simulink model "Turbine_State_Machine_Testrig_org"  (Simulink 10.0)
settings: Solver=ode45  StartTime=0.0  StopTime=20  MaxStep=1e-4  RelTol=1e-3  EnableMultiTasking=on
undefined symbols (not defined in the file): sigbuilder_block
libraries: Turbine_State_Machine_Lib x1
Description:
  | Copyright 2009-2017 The MathWorks, Inc. MathWorks, Inc.
settings Model: Creator=smiller  LastModifiedBy=bhisma
settings DataIOCC: LimitDataPoints=on  SignalLoggingSaveFormat=ModelDataLogs
settings OptimizationCC: ExpressionDepthLimit=2147483647
settings DebuggingCC: FcnCallInpInsideContextMsg=warning  AllowSymbolicDim=off  StateNameClashWarn=warning
settings SFSimCC: SimParseCustomCode=off
settings GRTTargetCC: GeneratePreprocessorConditionals=Disable all
settings ConfigComp: CovExternalEMLEnable=off  CovSFcnEnable=off

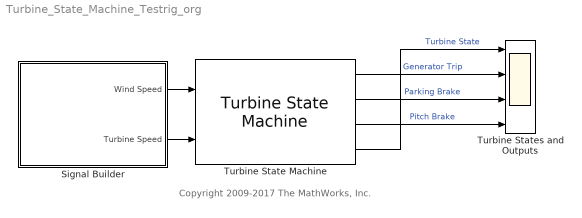
== system Turbine_State_Machine_Testrig_org ==
  note: Copyright 2009-2017 The MathWorks, Inc.
  Signal Builder : Subsystem  Tag=STV Subsys  LoadFcn=sigbuilder_block('load');  StartFcn=sigbuilder_block('start');  StopFcn=sigbuilder_block('stop');  ClipboardFcn=sigbuilder_block('clipboard');  mask(Sigbuilder block){tuvar=[0:10]}
      mask help: Sigbuilder GUI
      mask init:
      | if ~strcmp(get_param(bdroot(gcbh),'SimulationStatus'),'stopped') tuvar = sigbuilder_block('maskInit'); end
      settings: CopyFcn=sigbuilder_block('copy');  DeleteFcn=sigbuilder_block('delete');  ModelCloseFcn=sigbuilder_block('modelClose');  PreSaveFcn=sigbuilder_block('preSave');  PauseFcn=sigbuilder_block('pause')  ContinueFcn=sigbuilder_block('continue')  NameChangeFcn=sigbuilder_block('namechange');  OpenFcn=sigbuilder_block('open',[3 32.25 762 490.5 ]);  CloseFcn=sigbuilder_block('close');
      mask Display: plot(0, 0, 100, 100,[2, 2, 32, 32, 2], [68, 8, 8, 68, 68],[32, 2], [38, 38], [32, 19, 2],[53, 60, 44], [32, 17, 17, 2],[16, 16, 31, 31]);txt = getActiveGroup(gcbh);text(2, 100, txt,'verticalAlignment', 'top');
  Turbine State Machine : Turbine_State_Machine_Lib/Turbine State Machine
  Turbine States and Outputs : Scope  NumInputPorts=4
  wires:
  Turbine State Machine/4 -> Turbine States and Outputs/1  "Turbine State"
  Signal Builder/1(Wind Speed) -> Turbine State Machine/1
  Signal Builder/2(Turbine Speed) -> Turbine State Machine/2
  Turbine State Machine/1 -> Turbine States and Outputs/2  "Generator Trip"
  Turbine State Machine/2 -> Turbine States and Outputs/3  "Parking Brake"
  Turbine State Machine/3 -> Turbine States and Outputs/4  "Pitch Brake"

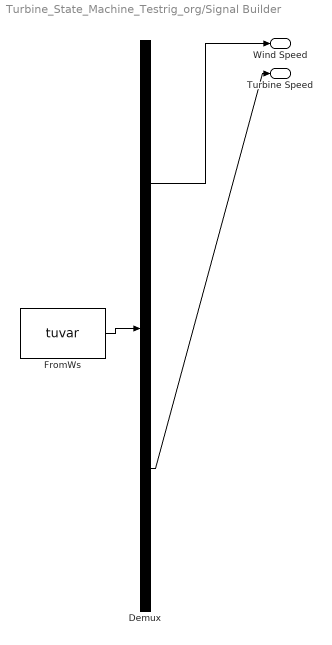
== system Turbine_State_Machine_Testrig_org/Signal Builder ==
  Demux : Demux  Tag=STV Demux  Outputs=2
  FromWs : FromWorkspace  Tag=STV FromWs  VariableName=tuvar  SampleTime=0  SigBuilderData=DataTag0  VnvData=DataTag1
      SigBuilderData=|
      | common.afterFinalStr = 'Extrapolate'
      | common.sampleTime = 0
      | dataSet(1).timeRange = [0 20]
      | dataSet(1).name = 'Simple Start and Stop'
      | dataSet(2).timeRange = [0 20]
      | dataSet(2).name = 'High Winds'
      | dataSet(3).timeRange = [0 20]
      | dataSet(3).name = 'Turbine Overspeed'
      | sbobj.Groups(1).Name = 'Simple Start and Stop'
      | sbobj.Groups(1).Signals(1).Name = 'Wind Speed'
      | sbobj.Groups(1).Signals(1).XData = [0 6 8.66 14 20]
      | sbobj.Groups(1).Signals(1).YData = [0 10 10 0 0]
      | sbobj.Groups(1).Signals(2).Name = 'Turbine Speed'
      | sbobj.Groups(1).Signals(2).XData = [0 4.42 4.42 6.46 10.02 16 20]
      | sbobj.Groups(1).Signals(2).YData = [0 0 0.37 1800 1800 0 0]
      | sbobj.Groups(2).Name = 'High Winds'
      | sbobj.Groups(2).Signals(1).Name = 'Wind Speed'
      | sbobj.Groups(2).Signals(1).XData = [0 4 6 8.66 20]
      | sbobj.Groups(2).Signals(1).YData = [0 10 10 22 22]
      | sbobj.Groups(2).Signals(2).Name = 'Turbine Speed'
      | sbobj.Groups(2).Signals(2).XData = [0 4.42 4.42 6.46 10.02 11.98 11.98 20]
      | sbobj.Groups(2).Signals(2).YData = [0 0 0.37 1800 1800 20 0 0]
      | sbobj.Groups(3).Name = 'Turbine Overspeed'
      | sbobj.Groups(3).Signals(1).Name = 'Wind Speed'
      | sbobj.Groups(3).Signals(1).XData = [0 4 6 8.66 14.85 20]
      | sbobj.Groups(3).Signals(1).YData = [0 10 10 12 12 12]
      | sbobj.Groups(3).Signals(2).Name = 'Turbine Speed'
      | sbobj.Groups(3).Signals(2).XData = [0 4.42 4.42 6.46 10.02 11.98 15.5 18.94 20]
      | sbobj.Groups(3).Signals(2).YData = [0 0 0.37 1800 1800 2200 2200 0 0]
  Wind Speed : Outport  Tag=STV Outport
  Turbine Speed : Outport  Tag=STV Outport  Port=2
  wires:
  Demux/1 -> Wind Speed/1
  FromWs/1 -> Demux/1
  Demux/2 -> Turbine Speed/1
